simulink model "app_VelocityMgr"  (R2016b)
settings: Solver=FixedStepDiscrete  StartTime=0.0  StopTime=1000  FixedStep=0.001  RelTol=1e-3  EnableMultiTasking=on
PreLoadFcn:
  | try
  |    tapas_types('load');
  | catch
  |   disp('TAPAS WARNING: Tapas Types could not be loaded ...');
  | end
  | 
  | try
  |   app_types('load');
  | catch
  |   currdir =pwd;
  |   try
  |     cd('..\app_types\');
  |     app_types('load');
  |     cd(currdir);
  |   catch
  |     try
  |        cd('..\..\app_types\');
  |        app_types('load');
  |        cd(currdir);
  |     catch
  |        cd(currdir);
  |        disp('TAPAS WARNING: Application Types could not be loaded ...');
  |     end
  |   end
  |   try
  |       clear currdir;
  |   catch
  |      %Do nothing
  |   end
  | end
settings Model: Creator=kmansour  LastModifiedBy=kmansour
settings DataIOCC: LimitDataPoints=on  SaveFormat=Array
settings OptimizationCC: LifeSpan=1
settings DebuggingCC: AllowSymbolicDim=off  SFUnexpectedBacktrackingDiag=warning  SFNoUnconditionalDefaultTransitionDiag=warning  SFExecutionAtInitializationDiag=none
settings HardwareCC: ProdBitPerPointer=32  ProdBitPerSizeT=32  ProdBitPerPtrDiffT=32  ProdLargestAtomicFloat=None  ProdIntDivRoundTo=Undefined  ProdEndianess=Unspecified  ProdWordSize=32  ProdHWDeviceType=32-bit Generic
settings ModelReferenceCC: ModelReferenceNumInstancesAllowed=Single  PropagateSignalLabelsOutOfModel=off
settings RTWCC: SystemTargetFile=ert.tlc  GenCodeOnly=on  TemplateMakefile=ert_default_tmf  Description=Embedded Coder  GenerateReport=on  CustomSourceCode="#include \"rte.h\""  IncludeHyperlinkInReport=on  LaunchReport=on  GenerateTraceInfo=on  GenerateTraceReport=on  GenerateTraceReportSl=on  GenerateTraceReportSf=on  GenerateTraceReportEml=on
settings CodeAppCC: IgnoreCustomStorageClasses=off  MaxIdLength=63
settings ERTTargetCC: GenerateSampleERTMain=on  ERTSrcFileBannerTemplate=tapas_code_template.cgt  ERTHdrFileBannerTemplate=tapas_code_template.cgt  ERTDataSrcFileTemplate=tapas_code_template.cgt  ERTDataHdrFileTemplate=tapas_code_template.cgt  ERTCustomFileTemplate=example_file_process.tlc  ConvertIfToSwitch=off  SuppressUnreachableDefaultCases=off
settings ConfigComp: CovMetricSettings=dw  CovHtmlReporting=on  CovSaveCumulativeToWorkspaceVar=on  CovSaveSingleToWorkspaceVar=on  CovExternalEMLEnable=off

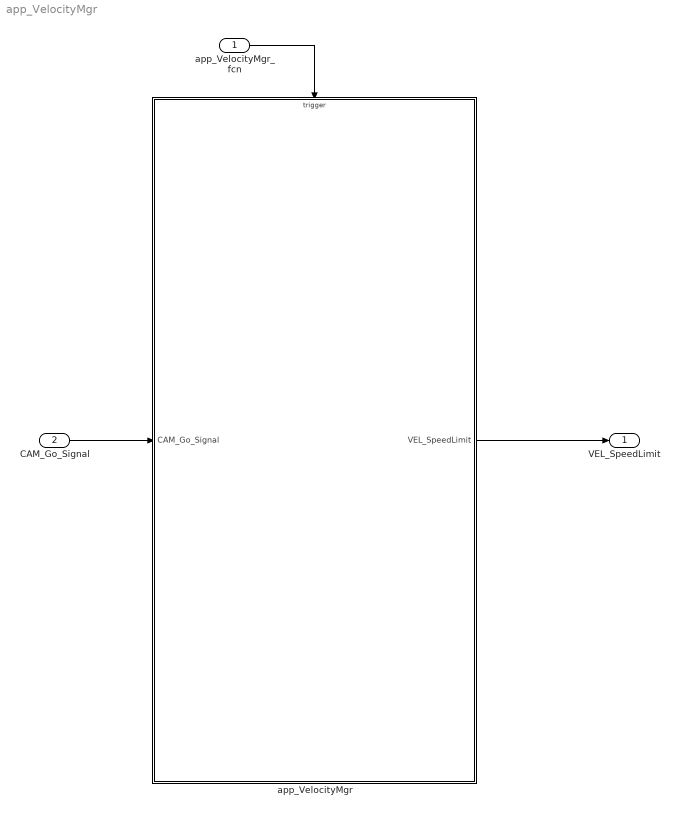
== system app_VelocityMgr ==
  app_VelocityMgr_fcn : Inport  SampleTime=10e-3  OutputFunctionCall=on
  CAM_Go_Signal : Inport  Port=2
  app_VelocityMgr : Subsystem
  VEL_SpeedLimit : Outport
  wires:
  app_VelocityMgr_fcn/1 -> app_VelocityMgr/Trigger
  CAM_Go_Signal/1 -> app_VelocityMgr/1(CAM_Go_Signal)
  app_VelocityMgr/1(VEL_SpeedLimit) -> VEL_SpeedLimit/1

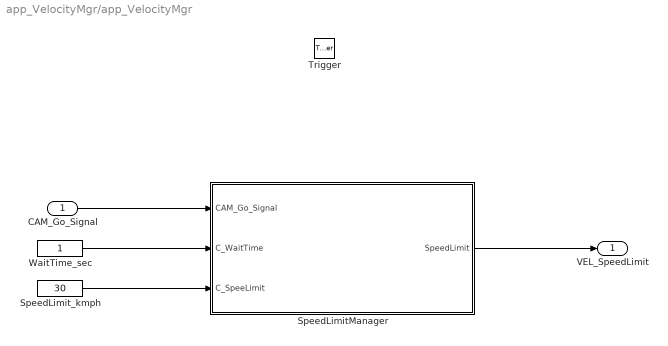
== system app_VelocityMgr/app_VelocityMgr ==
  CAM_Go_Signal : Inport
  Trigger : TriggerPort  TriggerType=function-call  VariantControl=Variant  SampleTimeType=periodic  SampleTime=-1  PortDimensions=1
  SpeedLimitManager : Stateflow chart  TreatAsAtomicUnit=on
  SpeedLimit_kmph : Constant  Value=30
  WaitTime_sec : Constant
  VEL_SpeedLimit : Outport
  wires:
  CAM_Go_Signal/1 -> SpeedLimitManager/1(CAM_Go_Signal)
  WaitTime_sec/1 -> SpeedLimitManager/2(C_WaitTime)
  SpeedLimit_kmph/1 -> SpeedLimitManager/3(C_SpeeLimit)
  SpeedLimitManager/1(SpeedLimit) -> VEL_SpeedLimit/1

== stateflow chart app_VelocityMgr/SpeedLimitManager ==
  state GO
    du:
    SpeedLimit = C_SpeeLimit;
  state STOP
    du:
    SpeedLimit = 0;
  state WAIT
    du:
    SpeedLimit = 0;
  (default) -> GO
  GO -> STOP : [CAM_Go_Signal == 0]
  (junction 7) -> STOP [order 2] : [CAM_Go_Signal == 0]
  STOP -> WAIT : [CAM_Go_Signal == 1]
  (junction 7) -> GO [order 1] : [CAM_Go_Signal == 1]
  WAIT -> (junction 7) : after(C_WaitTime,sec)
  data: CAM_Go_Signal input; C_WaitTime input; C_SpeeLimit input; SpeedLimit output
